simulink model "sampleModel1795"  (R2023a)
settings: Solver=VariableStepAuto  StartTime=0.0  StopTime=10.0  RelTol=1e-3
libraries: hdlsllib x5, simulink x5
settings Model: Creator=user1  LastModifiedBy=user1

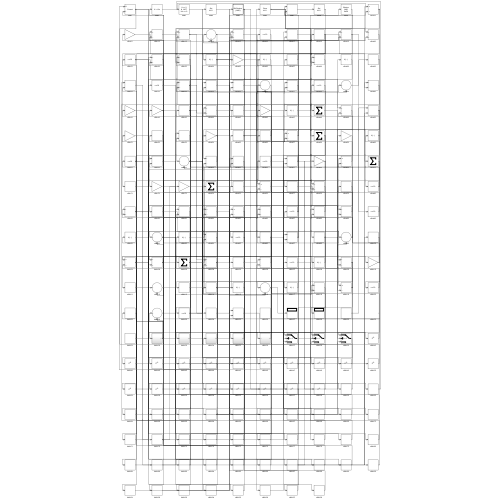
[thumbnail: Simulink's stored preview of the top-level diagram]
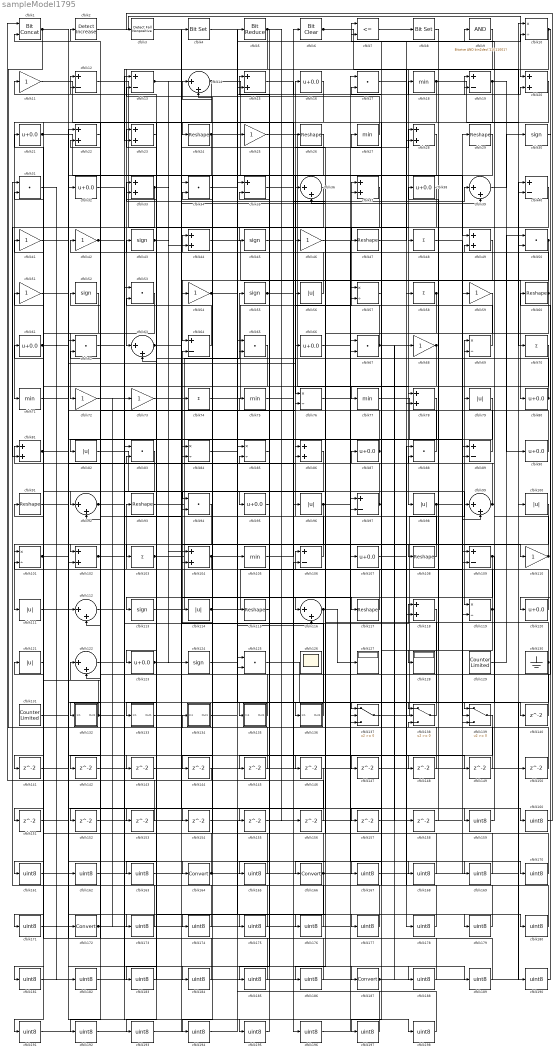
== system sampleModel1795 ==
  cfblk1 : hdlsllib/Logic and Bit Operations/Bit Concat  numInputs=2
  cfblk{10,57,69,76,84..85,101,119} (8 alike) : Product  Inputs=*/  RndMeth=Zero  SaturateOnIntegerOverflow=on
  cfblk{56,79,82,96,98,100,111,114,121} (9 alike) : Abs  SaturateOnIntegerOverflow=off
  cfblk{15,20,22..23,28,33,37,44,49,78,81,86,102,104,118} (15 alike) : Sum
  cfblk{48,58,70,74,103} (5 alike) : Sum  Inputs=+
  cfblk{18,27,71,75,77,105} (6 alike) : MinMax
  cfblk{12..13,19,35,40,64,89,97,106,109} (10 alike) : Sum  Inputs=+-
  cfblk{16,21,32,38,61,66,80,87,90,95,107,120,123} (13 alike) : Bias  Bias=0.0  SaturateOnIntegerOverflow=off
  cfblk{24,26,29,47,60,91,93,108,115,117} (10 alike) : Reshape
  cfblk{11,25,41..42,46,51,54,59,68,72..73,110} (12 alike) : Gain
  cfblk{14,36,39,63,92,99,112,116,122} (9 alike) : Sum  Inputs=|++
  cfblk{30,43,45,52,55,113,124} (7 alike) : Signum
  cfblk{17,31,34,50,53,62,65,67,83,88,94,125} (12 alike) : DotProduct  OutDataTypeStr=Inherit: Inherit via internal rule
  cfblk126 : Scope
      settings: Floating=on
  cfblk127 : Display
  cfblk128 : Display
  cfblk129 : hdlsllib/Sources/Counter Limited  uplimit=7  tsamp=-1
  cfblk130 : Ground
  cfblk131 : hdlsllib/Sources/Counter Limited  uplimit=7  tsamp=-1
  cfblk132 : Subsystem
      settings: LibrarySourceBlock=|
      | hdlsllib/Ports &
      | Subsystems/Subsystem
  cfblk133 : Subsystem
      settings: LibrarySourceBlock=|
      | hdlsllib/Ports &
      | Subsystems/Subsystem
  cfblk134 : Subsystem
      settings: LibrarySourceBlock=|
      | hdlsllib/Ports &
      | Subsystems/Subsystem
  cfblk135 : Subsystem
      settings: LibrarySourceBlock=|
      | hdlsllib/Ports &
      | Subsystems/Subsystem
  cfblk136 : Subsystem
      settings: LibrarySourceBlock=|
      | hdlsllib/Ports &
      | Subsystems/Subsystem
  cfblk137 : Switch  SaturateOnIntegerOverflow=off  InputSameDT=off
  cfblk138 : Switch  SaturateOnIntegerOverflow=off  InputSameDT=off
  cfblk139 : Switch  SaturateOnIntegerOverflow=off  InputSameDT=off
  cfblk{140..158} (19 alike) : Delay  SampleTime=1
  cfblk{159..163,165,167..171,173..186,188..198} (36 alike) : DataTypeConversion  OutDataTypeStr=uint8  SaturateOnIntegerOverflow=off  RndMeth=Floor
  cfblk{164,166,172,187} (4 alike) : DataTypeConversion  SaturateOnIntegerOverflow=off  RndMeth=Floor
  cfblk2 : simulink/Logic and Bit Operations/Detect Increase  vinit=0.0  OutDataTypeStr=boolean
      settings: LibrarySourceBlock=|
      | hdlsllib/Logic and Bit
      | Operations/Detect
      | Increase
  cfblk3 : hdlsllib/Logic and Bit Operations/Detect Fall Nonpositive  vinit=0  OutDataTypeStr=boolean
  cfblk4 : simulink/Logic and Bit Operations/Bit Set  iBit=0
      settings: LibrarySourceBlock=|
      | hdlsllib/Logic and Bit
      | Operations/Bit Set
  cfblk5 : hdlsllib/Logic and Bit Operations/Bit Reduce  mode=AND
  cfblk6 : simulink/Logic and Bit Operations/Bit Clear  iBit=0
      settings: LibrarySourceBlock=|
      | hdlsllib/Logic and Bit
      | Operations/Bit Clear
  cfblk7 : RelationalOperator  Operator=<=  OutDataTypeStr=boolean  InputSameDT=off
  cfblk8 : simulink/Logic and Bit Operations/Bit Set  iBit=0
      settings: LibrarySourceBlock=|
      | hdlsllib/Logic and Bit
      | Operations/Bit Set
  cfblk9 : simulink/Logic and Bit Operations/Bitwise Operator  logicop=AND  UseBitMask=on  BitMask=bin2dec('11011001')  BitMaskRealWorld=Stored Integer
      settings: LibrarySourceBlock=|
      | hdlsllib/Logic and Bit
      | Operations/Bitwise
      | Operator
  wires:
  cfblk9/1 -> cfblk98/1
  cfblk49/1 -> cfblk64/1
  cfblk129/1 -> cfblk50/1
  cfblk136/1(Out1) -> cfblk64/2
  cfblk43/1 -> cfblk124/1, cfblk123/1
  cfblk41/1 -> cfblk164/1
  cfblk52/1 -> cfblk72/1
  cfblk12/1 -> cfblk48/1
  cfblk30/1 -> cfblk116/1
  cfblk80/1 -> cfblk11/1, cfblk23/1
  cfblk98/1 -> cfblk110/1, cfblk191/1
  cfblk103/1 -> cfblk55/1, cfblk117/1
  cfblk22/1 -> cfblk92/1
  cfblk47/1 -> cfblk9/1
  cfblk137/1 -> cfblk69/1
  cfblk4/1 -> cfblk105/1
  cfblk109/1 -> cfblk113/1, cfblk139/1
  cfblk108/1 -> cfblk16/1
  cfblk10/1 -> cfblk120/1, cfblk23/2
  cfblk74/1 -> cfblk37/1
  cfblk40/1 -> cfblk47/1
  cfblk86/1 -> cfblk133/1(In1)
  cfblk25/1 -> cfblk78/1
  cfblk2/1 -> cfblk20/1
  cfblk48/1 -> cfblk89/1
  cfblk100/1 -> cfblk132/1(In1)
  cfblk29/1 -> cfblk76/1
  cfblk20/1 -> cfblk71/1
  cfblk70/1 -> cfblk102/1
  cfblk110/1 -> cfblk81/1, cfblk7/2
  cfblk5/1 -> cfblk63/1, cfblk95/1, cfblk156/1
  cfblk69/1 -> cfblk56/1
  cfblk75/1 -> cfblk39/1
  cfblk21/1 -> cfblk112/1, cfblk49/1
  cfblk19/1 -> cfblk77/1, cfblk90/1
  cfblk67/1 -> cfblk26/1, cfblk158/1
  cfblk120/1 -> cfblk38/1
  cfblk138/1 -> cfblk106/1
  cfblk123/1 -> cfblk74/1, cfblk28/1
  cfblk6/1 -> cfblk58/1, cfblk70/1, cfblk28/2
  cfblk95/1 -> cfblk135/1(In1)
  cfblk15/1 -> cfblk20/2
  cfblk33/1 -> cfblk81/2, cfblk44/2
  cfblk124/1 -> cfblk76/2
  cfblk68/1 -> cfblk171/1, cfblk176/1
  cfblk99/1 -> cfblk69/2, cfblk22/2
  cfblk114/1 -> cfblk29/1, cfblk116/2
  cfblk130/1 -> cfblk33/1, cfblk137/2
  cfblk89/1 -> cfblk57/1
  cfblk59/1 -> cfblk166/1
  cfblk62/1 -> cfblk187/1
  cfblk63/1 -> cfblk4/1, cfblk147/1, cfblk148/1
  cfblk117/1 -> cfblk93/1
  cfblk39/1 -> cfblk30/1
  cfblk8/1 -> cfblk128/1
  cfblk102/1 -> cfblk12/1, cfblk177/1
  cfblk28/1 -> cfblk102/2
  cfblk87/1 -> cfblk15/1, cfblk12/2
  cfblk131/1 -> cfblk75/1
  cfblk36/1 -> cfblk63/2
  cfblk44/1 -> cfblk80/1
  cfblk82/1 -> cfblk119/1
  cfblk58/1 -> cfblk97/2, cfblk157/1
  cfblk7/1 -> cfblk8/1
  cfblk34/1 -> cfblk136/1(In1)
  cfblk18/1 -> cfblk40/2, cfblk103/1, cfblk45/1, cfblk141/1
  cfblk55/1 -> cfblk57/2, cfblk19/2
  cfblk81/1 -> cfblk61/1, cfblk84/2, cfblk143/1
  cfblk54/1 -> cfblk10/2, cfblk174/1
  cfblk27/1 -> cfblk13/2
  cfblk61/1 -> cfblk89/2, cfblk182/1
  cfblk45/1 -> cfblk6/1
  cfblk105/1 -> cfblk37/2
  cfblk101/1 -> cfblk86/2, cfblk149/1
  cfblk90/1 -> cfblk36/1
  cfblk50/1 -> cfblk139/2, cfblk186/1
  cfblk94/1 -> cfblk111/1
  cfblk57/1 -> cfblk27/1
  cfblk92/1 -> cfblk94/2, cfblk180/1
  cfblk79/1 -> cfblk82/1
  cfblk104/1 -> cfblk19/1, cfblk101/2
  cfblk73/1 -> cfblk99/1
  cfblk71/1 -> cfblk66/1
  cfblk132/1(Out1) -> cfblk118/1, cfblk51/1, cfblk21/1
  cfblk112/1 -> cfblk137/1
  cfblk14/1 -> cfblk18/1, cfblk24/1
  cfblk31/1 -> cfblk172/1
  cfblk84/1 -> cfblk115/1
  cfblk1/1 -> cfblk134/1(In1), cfblk137/3, cfblk195/1
  cfblk64/1 -> cfblk33/2
  cfblk42/1 -> cfblk94/1, cfblk142/1
  cfblk133/1(Out1) -> cfblk39/2
  cfblk60/1 -> cfblk43/1, cfblk119/2
  cfblk88/1 -> cfblk14/2
  cfblk77/1 -> cfblk109/1
  cfblk113/1 -> cfblk86/1
  cfblk97/1 -> cfblk7/1, cfblk87/1
  cfblk56/1 -> cfblk2/1
  cfblk119/1 -> cfblk36/2, cfblk49/2, cfblk167/1
  cfblk106/1 -> cfblk52/1
  cfblk93/1 -> cfblk15/2
  cfblk13/1 -> cfblk109/2, cfblk104/1
  cfblk135/1(Out1) -> cfblk44/1
  cfblk24/1 -> cfblk78/2, cfblk10/1, cfblk25/1, cfblk163/1
  cfblk96/1 -> cfblk101/1, cfblk112/2, cfblk108/1
  cfblk116/1 -> cfblk127/1, cfblk144/1
  cfblk134/1(Out1) -> cfblk138/1
  cfblk11/1 -> cfblk96/1
  cfblk38/1 -> cfblk118/2
  cfblk66/1 -> cfblk140/1
  cfblk140/1 -> cfblk1/2
  cfblk142/1 -> cfblk106/2
  cfblk143/1 -> cfblk40/1
  cfblk144/1 -> cfblk1/1
  cfblk139/1 -> cfblk145/1
  cfblk145/1 -> cfblk14/1
  cfblk37/1 -> cfblk146/1
  cfblk147/1 -> cfblk138/2
  cfblk148/1 -> cfblk104/2
  cfblk149/1 -> cfblk34/1
  cfblk150/1 -> cfblk88/2
  cfblk121/1 -> cfblk151/1
  cfblk16/1 -> cfblk152/1
  cfblk152/1 -> cfblk99/2
  cfblk23/1 -> cfblk153/1
  cfblk153/1 -> cfblk22/1
  cfblk91/1 -> cfblk154/1
  cfblk118/1 -> cfblk155/1
  cfblk155/1 -> cfblk67/2
  cfblk156/1 -> cfblk92/2
  cfblk158/1 -> cfblk138/3
  cfblk3/1 -> cfblk159/1
  cfblk159/1 -> cfblk79/1
  cfblk107/1 -> cfblk160/1
  cfblk160/1 -> cfblk3/1
  cfblk53/1 -> cfblk161/1
  cfblk161/1 -> cfblk5/1
  cfblk51/1 -> cfblk162/1
  cfblk162/1 -> cfblk53/1
  cfblk163/1 -> cfblk53/2
  cfblk164/1 -> cfblk139/3, cfblk84/1, cfblk107/1, cfblk50/2
  cfblk78/1 -> cfblk165/1
  cfblk165/1 -> cfblk41/1
  cfblk166/1 -> cfblk114/1, cfblk13/1, cfblk183/1
  cfblk167/1 -> cfblk59/1
  cfblk46/1 -> cfblk168/1
  cfblk168/1 -> cfblk42/1
  cfblk76/1 -> cfblk169/1
  cfblk169/1 -> cfblk46/1
  cfblk32/1 -> cfblk170/1
  cfblk170/1 -> cfblk34/2
  cfblk171/1 -> cfblk32/1
  cfblk172/1 -> cfblk97/1, cfblk73/1
  cfblk141/1 -> cfblk173/1
  cfblk173/1 -> cfblk31/1
  cfblk174/1 -> cfblk31/2
  cfblk85/1 -> cfblk175/1
  cfblk175/1 -> cfblk91/1
  cfblk176/1 -> cfblk85/1
  cfblk177/1 -> cfblk85/2
  cfblk17/1 -> cfblk178/1
  cfblk178/1 -> cfblk88/1
  cfblk154/1 -> cfblk179/1
  cfblk179/1 -> cfblk17/1
  cfblk180/1 -> cfblk17/2
  cfblk83/1 -> cfblk181/1
  cfblk181/1 -> cfblk150/1
  cfblk182/1 -> cfblk83/1
  cfblk183/1 -> cfblk83/2
  cfblk122/1 -> cfblk184/1
  cfblk184/1 -> cfblk121/1
  cfblk115/1 -> cfblk185/1
  cfblk185/1 -> cfblk122/1
  cfblk186/1 -> cfblk122/2
  cfblk187/1 -> cfblk100/1, cfblk68/1
  cfblk111/1 -> cfblk188/1
  cfblk188/1 -> cfblk62/1
  cfblk151/1 -> cfblk189/1
  cfblk189/1 -> cfblk62/2
  cfblk125/1 -> cfblk190/1
  cfblk190/1 -> cfblk60/1
  cfblk191/1 -> cfblk125/1
  cfblk146/1 -> cfblk192/1
  cfblk192/1 -> cfblk125/2
  cfblk65/1 -> cfblk193/1
  cfblk193/1 -> cfblk54/1
  cfblk26/1 -> cfblk194/1
  cfblk194/1 -> cfblk65/1
  cfblk195/1 -> cfblk65/2
  cfblk35/1 -> cfblk196/1
  cfblk196/1 -> cfblk67/1
  cfblk157/1 -> cfblk197/1
  cfblk197/1 -> cfblk35/1
  cfblk72/1 -> cfblk198/1
  cfblk198/1 -> cfblk35/2

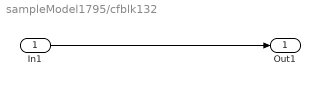
== system sampleModel1795/cfblk132 ==
  In1 : Inport
  Out1 : Outport
  wires:
  In1/1 -> Out1/1

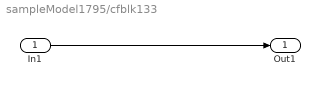
== system sampleModel1795/cfblk133 ==
  In1 : Inport
  Out1 : Outport
  wires:
  In1/1 -> Out1/1

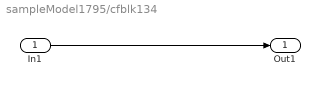
== system sampleModel1795/cfblk134 ==
  In1 : Inport
  Out1 : Outport
  wires:
  In1/1 -> Out1/1

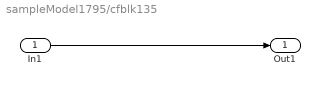
== system sampleModel1795/cfblk135 ==
  In1 : Inport
  Out1 : Outport
  wires:
  In1/1 -> Out1/1

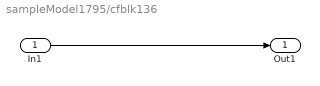
== system sampleModel1795/cfblk136 ==
  In1 : Inport
  Out1 : Outport
  wires:
  In1/1 -> Out1/1
